simulink model "follow_blob"  (R2024b)
settings: Solver=VariableStepAuto  StartTime=0.0  StopTime=inf  RelTol=1e-3
libraries: robotlib x6
settings Model: Creator=ABHIRAJ  LastModifiedBy=ABHIRAJ

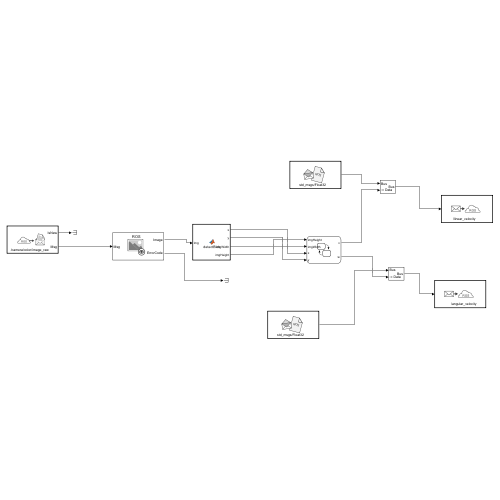
[thumbnail: Simulink's stored preview of the top-level diagram]
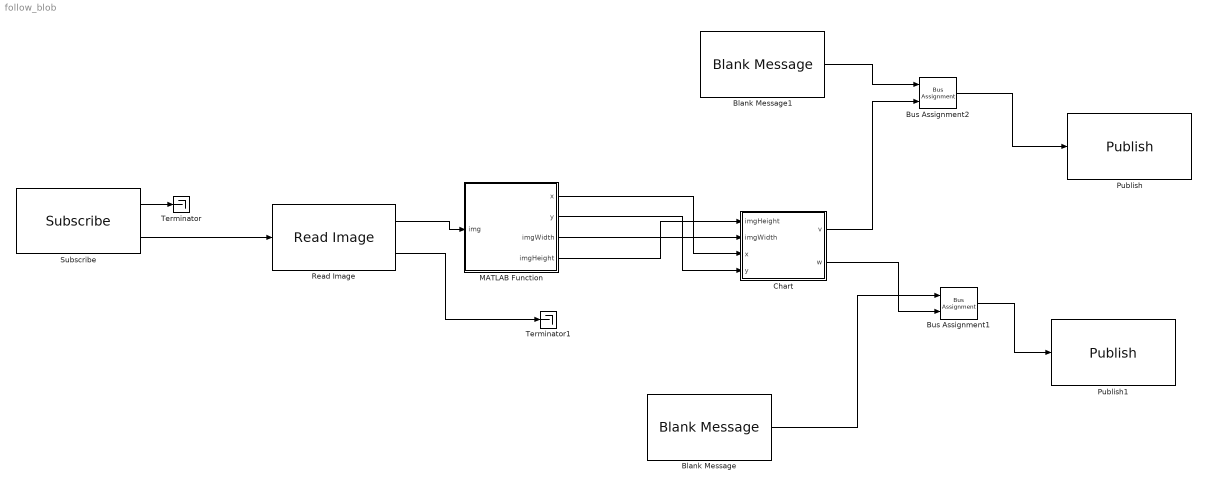
== system follow_blob ==
  Blank Message : robotlib/Blank Message  messageClass=Message  entityType=std_msgs/Float32  messageType=std_msgs/Float32  SampleTime=inf  legacyBusStruct=off
  Blank Message1 : robotlib/Blank Message  messageClass=Message  entityType=std_msgs/Float32  messageType=std_msgs/Float32  SampleTime=inf  legacyBusStruct=off
  Bus Assignment1 : BusAssignment  AssignedSignals=Data
  Bus Assignment2 : BusAssignment  AssignedSignals=Data
  Chart : Stateflow chart  TreatAsAtomicUnit=on
  MATLAB Function : MATLAB Function  TreatAsAtomicUnit=on
  Publish : robotlib/Publish  topicSource=Select from ROS network  topic=/linear_velocity  messageType=std_msgs/Float32  legacyBusStruct=off  messageQueueLength=1
  Publish1 : robotlib/Publish  topicSource=Select from ROS network  topic=/angular_velocity  messageType=std_msgs/Float32  legacyBusStruct=off  messageQueueLength=1
  Read Image : robotlib/Read Image  MaximumImageSize=[ 480, 640 ]  ImageEncoding=rgb8  ShowAlphaOutput=off  ShowErrorCodeOutput=on  VariableSizeOutputs=off
  Subscribe : robotlib/Subscribe  topicSource=Select from ROS network  topic=/camera/color/image_raw  messageType=sensor_msgs/Image  SampleTime=-1  legacyBusStruct=off  messageQueueLength=1
  Terminator : Terminator
  Terminator1 : Terminator
  wires:
  MATLAB Function/1(x) -> Chart/3(x)
  MATLAB Function/2(y) -> Chart/4(y)
  MATLAB Function/3(imgWidth) -> Chart/2(imgWidth)
  MATLAB Function/4(imgHeight) -> Chart/1(imgHeight)
  Subscribe/1 -> Terminator/1
  Subscribe/2 -> Read Image/1
  Read Image/1 -> MATLAB Function/1(img)
  Read Image/2 -> Terminator1/1
  Blank Message/1 -> Bus Assignment1/1
  Chart/2(w) -> Bus Assignment1/2
  Bus Assignment1/1 -> Publish1/1
  Blank Message1/1 -> Bus Assignment2/1
  Chart/1(v) -> Bus Assignment2/2
  Bus Assignment2/1 -> Publish/1

== matlab function follow_blob/MATLAB Function ==
  data: x output; img input; y output; imgWidth output; imgHeight output
function [x, y, imgWidth, imgHeight] = detectBlob(img) 
    % Get the size of the image (height, width)
    [imgHeight, imgWidth, ~] = size(img);

    I = img;

% Define thresholds for channel 1 based on histogram settings
    channel1Min = 0.000;
    channel1Max = 65.000;

% Define thresholds for channel 2 based on histogram settings
    channel2Min = 0.000;
    channel2Max = 125.000;

% Define thresholds for channel 3 based on histogram settings
    channel3Min = 52.000;
    channel3Max = 255.000;

% Create mask based on chosen histogram thresholds
    sliderBW = (I(:,:,1) >= channel1Min ) & (I(:,:,1) <= channel1Max) & ...
        (I(:,:,2) >= channel2Min ) & (I(:,:,2) <= channel2Max) & ...
        (I(:,:,3) >= channel3Min ) & (I(:,:,3) <= channel3Max);

    % Perform blob analysis to detect the blobs
    hBlob = vision.BlobAnalysis('MinimumBlobArea', 30000, 'MaximumBlobArea', 500000);

    % Run blob analysis on the binary image
    [Area, Centroid] = step(hBlob, sliderBW);

    % Find the largest blob (assuming it's the target object)
     if ~isempty(Area)
        % Output the X, Y coordinates of the centroid
        x = Centroid(1);
        y = Centroid(2);
    else
        % If no blob is detected, return NaN values
        x = NaN;
        y = NaN;
    end
        % If no blob is detected, return NaN values
       
end

== stateflow chart follow_blob/Chart ==
  state Tracking
    entry,during:
    [v,  w] = calculateVelocity(x, y, imgWidth, imgHeight);
  state Waiting
    entry:
    v = 0;
    w = 0;
  state Seeking
    entry:
    v = 0;
    w = 0.3;
  (default) -> Tracking
  Tracking -> Waiting : [isnan(x) || isnan(y)]
  Seeking -> Tracking : [~isnan(x) && ~isnan(y)]
  Waiting -> Seeking : after(4, sec)
  data: x function_input; y function_input; imgWidth function_input; imgHeight function_input; v function_output; w function_output; imgHeight input; imgWidth input; x input; y input; v output; w output
  function [v, w] = calculateVelocity(x, y, imgWidth, imgHeight):
    | function [v, w] = calculateVelocity(x, y, imgWidth, imgHeight)
    |     % Call the external function headingCorrection.m
    |     [v, w] = calcVel(x, y, imgWidth, imgHeight)
    | end
